simulink library "GTMLE_Library"  (R2014a)
settings: Solver=ode45  StartTime=0.0  StopTime=10.0  RelTol=1e-3
undefined symbols (not defined in the file or in its folder): CCP, DiscIntNeverNeededParam, DPos_test, sample_time, TData_test
undefined symbols (not defined in the file): MCP, steadydata
libraries: simulink x10, GTMLE_Library x2, discretizing x1
(part 1 of 2)
settings Model: CovSFcnEnable=on  Creator=Esrod  LastModifiedBy=Shubo

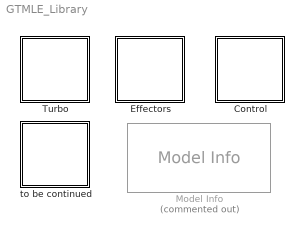
== system GTMLE_Library ==
  Control : Subsystem
  Effectors : Subsystem
  Model Info : simulink/Model-Wide Utilities/Model Info  Commented=on  InitialBlockCM=无  BlockCM=none  Frame=on  DisplayStringWithTags=|  HorizontalTextAlignment=Center  LeftAlignmentValue=0.5  SourceBlockDiagram=GTMLE_Library  TagMaxNumber=20
      | Model Info
      | %<ModifiedBy>
      | %<ModifiedDate>
      | %<ModifiedComment>
      | %<ModelVersion>
  Turbo : Subsystem
  to be continued : Subsystem

== system GTMLE_Library/Control ==
  ABControl : Subsystem  mask{CNST=CCP.CNST, PLA_TO=CCP.PLA_TO, PLA_MAX=CCP.PLA_MAX}
  Acc N1dot : Subsystem
  Acc Plan : Subsystem
  Static Control : Subsystem  mask{PLA_idle=CCP.PLA_idle, PLA_TO=CCP.PLA_TO, N1cor_TO=CCP.N1cor_TO*0.98, N1cor_idle=CCP.N1cor_idle}
  anti_windup : Subsystem

== system GTMLE_Library/Effectors ==
  DesignTools : Subsystem  InitFcn=load( 'resource/SS_Tool_result' );  mask{T4res=1700, SMres=20, n2_tab=steadydata(:,9), n2_Wfmin=steadydata(:,10)*0.7, kci=1e-4, accordec=2, statedata=[steadydata(:,10) steadydata(:,8) steadydata(:,9)]}
      mask prompts: T4res "T4resForAcc (K)"; SMres "SMresForAcc (%)"; n2_tab "n2_tab (rpm)"; n2_Wfmin "WfminForDec (kg/s)"; kci "kci (-)"; accordec "(1)ForAccPlan(2)ForDecPlan"
  Display_out : Subsystem
  Iterative NR Solver w JacobianCalc : Subsystem  mask(T-MATS: Iterative NR Solver w Jacobian Calc Library Block){SJac_Per_M=MCP.Solve.NR_Per_M(1:6,1), SNR_IC_M=MCP.Solve.NR_IC(1:6,1), SNR_DX_M=0.1, SJacobianAttempts_M=20, Cond_Limits_M=MCP.Solve.Cond_Limits_M}
      mask prompts: SJac_Per_M "SJac_Per_M - Jacobian Perturbation size (frac) (nx1)"; SNR_IC_M "SNR_IC_M - Newton Raphson Initial Conditions (nx1)"; SNR_DX_M "SNR_DX_M - Newton Raphson delta x limiter (%) (1x1)"; SJacobianAttempts_M "SJacobianAttempts_M - Newton Raphson attempts before the Jacobian recalculation (1x1)"; Cond_Limits_M "Cond_Limits_M - Iteration Conditions Limits (nx1 or 1x1)"
      mask help:
      | The Iterative Newton Raphson Solver with Jacobian Calculator block will
      | supply the inputs to iteratively drive the outputs of a system to zero.
      |
      | This will be performed in three steps.
      | 1) Jabobian calculator sends Perturbations to the plant then calculates the plant
      | Jacboian based on the system response
      | 2) The Newton Raphson will use the inverse of the Jacobian to iteratively step the
      | system toward solution.
      | 3) Once the solution has satisfied the conditions the Newton Raphson is shut off.
      |
      | This module is designed for dynamic systems and should be paired with
      | a "do... while" block in Simulink. The "do...while" block and this module
      | should both be located in the same subsystem as the plant that is to be solved for.
      mask Help: web(which('Solver_TMATS_INRSwJC.html'),'-helpbrowser')
  LoadTestData : Subsystem  mask{TData_test=TData_test, DPos_test=DPos_test}
  Mixer_Ades_calc : Subsystem  mask{Mades1=0.4, Mades2=0.451238}
      mask prompts: Mades1 "Core entry Mach in design condition"; Mades2 "Duct entry Mach in design condition"
  Performance : Subsystem
  SStool : Subsystem  StopFcn=|  mask{Wf_init=1.279, Wf_plan=[1 0.9 0.8 0.6 0.5 0.15], Cond_Limits_M=0.00001}
      | steadydata = importdata( 'resource/SS_Tool_Result.txt' );
      | save resource/SS_Tool_Result steadydata;                 
      | clearvars steadydata;                                    
      | delete( 'resource/SS_Tool_Result.txt' );

== system GTMLE_Library/Turbo ==
  Ambient : Subsystem
  Burner : Subsystem  mask(GTML_E: Burner Library Block){Eff_des=MCP.Buner.Eff_des, dpbur=MCP.Buner.dpbur, PtIn_des=MCP.Buner.PtIn_des, WIn_des=MCP.Buner.WIn_des, TtIn_des=MCP.Buner.TtIn_des, Volume=0.03, FuelType=Kerosene, TtIn_fuel=MCP.Buner.TtIn_fuel, LHV=MCP.Buner.LHV, FixEff=Constant Efficiency, CNST=MCP.Buner.CNST, Load_tab=MCP.Buner.Load_tab, Eff_tab=MCP.Buner.Eff_tab}
      mask prompts: Eff_des "Eff - Burner Efficiency"; dpbur "dpbur - Normalized Burner deltaP"; PtIn_des "<PtIn_des:kPa> - PtIn in design condition"; WIn_des "<WIn_des:kg/s> - WtIn in design condition"; TtIn_des "<TtIn_des:K> - TtIn in design condition"; Volume "Volume: m^3"; FuelType "Fuel type"; TtIn_fuel "<TtIn_fuel:K>"; LHV "<LHV:J/kg> - Fuel Lower Heating Value"; FixEff "Constant combustion efficiency"; Load_tab "Table of combustion load"; Eff_tab "Table of combustion efficiency"
      mask help: This block simulates the performance of a burner using basic thermodynamic equations and properties.
      mask TypeOptions FuelType: Kerosene | Nature Gas
      mask TypeOptions FixEff: Constant Efficiency | Using Characteristic Map
  Compressor : Subsystem  mask{CNST=MCP.Comp.CNST, N_tab=MCP.Comp.N_tab, Beta_tab=MCP.Comp.Beta_tab, Pi_tab=MCP.Comp.Pi_tab, Wcor_tab=MCP.Comp.Wcor_tab, Eta_tab=MCP.Comp.Eta_tab, CustBldsPlan=[0;0;0], FBldsPlan=[0;0;0], WcSurgeVec=MCP.Comp.WcSurgeVec, PRSurgeVec=MCP.Comp.PRSurgeVec}
  Duct : Subsystem  mask(Untitled: Duct Library Block){CNST=[101.325 288.15], sigma_des=0.8688, PtIn_des=292.164, WIn_des=35.22685, TtIn_des=430.59982}
      mask prompts: sigma_des "sigma_des - Rel. total pressure recovery coefficient"; PtIn_des "PtIn_des - PtIn in design condition"; WIn_des "WIn_des - WIn in design condition"; TtIn_des "TtIn_des - TtIn in design condition"
      mask help: This block simulates the performance of a duct using basic fluid dynamic equations and properties.
  Fan : Subsystem  mask{BPRdes=5.05, Cf=0}
  Heat Soakage : Subsystem  VariantControl=Variant1  mask(Heat Soakage){FCdes=MCP.Hpt.FC_des, Cpdes=MCP.Hpt.Cp_des, Wdes=MCP.Hpt.W_des, Aht=MCP.Hpt.Aht, Ck=MCP.Hpt.Ck, Mm=MCP.Hpt.Mm, Cm=MCP.Hpt.Cm, Ct=MCP.Hpt.Ct, x=MCP.Hpt.x}
      mask prompts: FCdes "FCdes[W/m^2 K]--Film coefficient"; Cpdes "Cpdes[J/kg K]--The gas specific heat in the design point"; Wdes "Wdes[kg/s]--Mass flow in the design point"; Aht "Aht[m^2]--Effective contact surface"; Ck "Ck[-] --A corrected factor for K"; Mm "Mm[kg]--Material effective mass"; Cm "Cm[J/kg K]--Material specific heat component material"; Ct "Ct[-]--A corrected factor for Tau"; x "x[-]--power,0~1"
      mask help:
      | K = Ck * FCdes * Aht * W^(x-1) / Cpdes / Wdes^x
      | Tau_inv = Ct * K * W * Cp / Cm / Mm
      | where Ct and Ck are corrected factors.
      | dTm/dt = Tau_inv * (Tg_ideal - Tm)
      | Tg_real = (1-K) * Tg_ideal + K * Tm
      mask Help:
      | Uht = 1/((1/FC)+(leff/km)) = FC when material thermal conductivity is not taken into account.
      | The material temperature dynamic response is a 1st order response following the equation:
      | 
      | Q =  Uht*Aht*(Tg_ideal-Tm)
      | 
      | FC is the film coefficient, calculated from
      | 
      | FC = FCdes*Cp/CPdes * (W/Wdes)^x
      | 
      | with FCdes as a user specified film coefficient in the design point. Cpdes and
      | Wdes are the gas specific heat and mass flow calculated for DP and Cp and
      | W the OD calculated values.
      | x = 0~1.
      | The average material temperature Tm is calculated by integrating:
      | 
      | dTm/dt = Q / (Cm*Mm)
      | 
      | Initial value for Tm is the steady state gas temperature. Since heat flow is
      | assumed to be proportional to the difference between gas and material temperature
      | the material temperature Tm follows the gas temperature Tg_ideal with a first
      | order lag.
      | The time constant is determined by:
      | 
      | Tau = Cm*Mm / (Uht*Aht)
      | 
      | The real gas temperature Tg_real is calculated by:
      | 
      | Tg_real = Tg_ideal - Q/W*Cp = (1-K) * Tg_ideal + K * Tm
      | 
      | with K = Ck * Uhtdes * Aht * W^(x-1) / Cpdes / Wdes^x
      | 
      | Symbols ---------- Description --------------------------------  Parameter name
      | Tm --------------- average material temperature
      | Tg_real --------------- average gas temperature
      | Aht -------------- effective contact surface -------------- Heat soak A
      | Cm --------------- specific heat component material ------- Heat soak Cp
      | Mm --------------- Effective mass ------------------------- Heat soak mass
      | Uht -------------- Heat transfer coefficient -------------- Uhsoak
      | Leff ------------- effective length heat flow transport --- Heat soak Leff
      | km --------------- material thermal conductivity ---------- Heat soak k
      | FC --------------- Film coefficient ----------------------- Heat soak film coefficient
      | W ---------------- Gas mass flow
      | Cp --------------- Gas specific heat
  Inlet : Subsystem  mask{sigma_inlet_des=MCP.Inlet.sigma}
  Mixer : Subsystem  mask(GTML_E: Mixer Library Block){Ades1=0.16, Ades2=0.18}
      mask prompts: Ades1 "<Acore_des:m^2> - Design core area"; Ades2 "<Aduct_des:m^2> - Design duct area"
      mask help: This block simulates the performance of a mixer.
  Nozzle : Subsystem  mask{CD=MCP.Ductnozzle.CD, CV=MCP.Ductnozzle.CV, CX=MCP.Ductnozzle.CX}
  Shaft : Subsystem  mask{J=MCP.Lowshaft.J, eta=MCP.Lowshaft.eta}
      mask prompts: J "<J:kg*m^2>"; eta "<ETAmech:->"
  Turbine : Subsystem  mask{CNST=MCP.Hpt.CNST, N_tab=MCP.Hpt.N_tab, Pi_tab=MCP.Hpt.Pi_tab, Wcor_tab=MCP.Hpt.Wcor_tab, Eta_tab=MCP.Hpt.Eta_tab, CoolingPlan=MCP.Hpt.CoolingPlan, FuelType=Kerosene}
      mask prompts: FuelType "Fuel type"
      mask TypeOptions FuelType: Kerosene | Nature Gas

== system GTMLE_Library/to be continued ==

== system GTMLE_Library/Control/ABControl ==
  PLA : Inport
  P2 : Inport  Port=2
  T2 : Inport  Port=3
  Divide : Product  Inputs=*/
  PLA_MAX : Constant  Value=PLA_MAX
  PLA_TO : Constant  Value=PLA_TO
  Product : Product
  Saturation : Saturate  UpperLimit=CCP.PLA_MAX  LowerLimit=CCP.PLA_TO
  Subsystem : Subsystem
  Sum : Sum  Inputs=|+-
  Sum1 : Sum  Inputs=|-+
  Wf_max : Constant  Value=CCP.AB.Wf_max
  Wf_ab : Outport
  wires:
  Saturation/1 -> Sum/1
  Wf_max/1 -> Subsystem/1(Wfmax)
  T2/1 -> Subsystem/3(T2)
  P2/1 -> Subsystem/2(P2)
  Subsystem/1(Wfmaxcor) -> Product/2
  Product/1 -> Wf_ab/1
  Divide/1 -> Product/1
  Sum1/1 -> Divide/2
  Sum/1 -> Divide/1
  PLA_MAX/1 -> Sum1/2
  PLA_TO/1 -> Sum/2, Sum1/1
  PLA/1 -> Saturation/1

== system GTMLE_Library/Control/Acc N1dot ==
  N1 : Inport
  Flag : Inport  Port=2
  Wf_initial : Inport  Port=3
  P2 : Inport  Port=4
  T2 : Inport  Port=5
  N2 : Inport  Port=6
  PI1 : Subsystem
  throttle plan : Subsystem
  WF_acc : Outport
  wires:
  N1/1 -> PI1/3(N1)
  T2/1 -> PI1/6(T2), throttle plan/3(T2)
  P2/1 -> PI1/5(P2), throttle plan/2(P2)
  Wf_initial/1 -> PI1/4(Wf_initial)
  N2/1 -> throttle plan/1(N2)
  Flag/1 -> PI1/2(Flag)
  throttle plan/1(" err_N2dot") -> PI1/1(y)
  PI1/1(Wf ndot) -> WF_acc/1

== system GTMLE_Library/Control/Acc Plan ==
  Ps3 : Inport
  N2 : Inport  Port=2
  T2 : Inport  Port=3
  1-D Lookup Table : Lookup_n-D  NumberOfTableDimensions=1  BreakpointsForDimension1=CCP.AccPlan.N2cor_Tab  Table=CCP.AccPlan.Wfcor_Tab  RndMeth=Simplest  InputSameDT=on
  Divide : Product  Inputs=*/
  Gain : Gain  Gain=1e-3
  Product : Product  RndMeth=Zero
  Product1 : Product  RndMeth=Zero
  a : Fcn  Expr=sqrt(288.15/u(1))
  Wfacc : Outport
  wires:
  1-D Lookup Table/1 -> Divide/1
  N2/1 -> Product/1
  Gain/1 -> Product1/2
  Product1/1 -> Wfacc/1
  Ps3/1 -> Gain/1  "kPa"
  Divide/1 -> Product1/1
  Product/1 -> 1-D Lookup Table/1
  a/1 -> Divide/2, Product/2
  T2/1 -> a/1

== system GTMLE_Library/Control/Static Control ==
  N1 : Inport
  PLA : Inport  Port=2
  T2 : Inport  Port=3
  P2 : Inport  Port=4
  Wf_initial : Inport  Port=5
  Flag : Inport  Port=6
  " " : Subsystem
  Display : Display
  Display1 : Display
  N1_cor : Subsystem
  Subsystem : Subsystem
  Sum : Sum  Inputs=|+-  SaturateOnIntegerOverflow=on
  Wfs : Outport
  wires:
  Flag/1 -> " "/6(Flag)
  Wf_initial/1 -> " "/5(Wf_initial)
  P2/1 -> " "/4(P2)
  T2/1 -> N1_cor/2(T2), " "/3(T2)
  PLA/1 -> Subsystem/1(PLA)
  Sum/1 -> " "/1(N1_eer)
  N1_cor/1(N1) -> Display/1, Sum/1
  Subsystem/1(N1cor) -> N1_cor/1(N1cor)
  " "/1(Wf) -> Wfs/1
  N1/1 -> Display1/1, " "/2(N1), Sum/2

== system GTMLE_Library/Control/anti_windup ==
  note: This block is for anti_windup.
      | Flag is for set point control, and the value of 1 represents to freeze the integral term, 0 to unfreeze the integral term.
      |  Flag2 is for acc. of N2dot control, and the value of 0 represents to freeze the integral term, 1 to unfreeze the integral term
      | Flag3 is for dec. of N2dot control, and the value of 0 represents to freeze the integral term, 1 to unfreeze the integral term
  set_point_Wf : Inport
  acc : Inport  Port=2
  acc_N2dot : Inport  Port=3
  dec : Inport  Port=4
  dec_N2dot : Inport  Port=5
  MinFcn : MATLAB Function  TreatAsAtomicUnit=on
  flag : Outport
  flag2 : Outport  Port=2
  Wf_above_idle : Outport  Port=3
  flag3 : Outport  Port=4
  wires:
  MinFcn/4(flag3) -> flag3/1
  MinFcn/2(flag) -> flag/1
  dec_N2dot/1 -> MinFcn/5(dec_N2dot)
  dec/1 -> MinFcn/3(dec)
  MinFcn/1(choose) -> Wf_above_idle/1
  MinFcn/3(flag2) -> flag2/1
  acc/1 -> MinFcn/2(acc)
  acc_N2dot/1 -> MinFcn/4(acc_N2dot)
  set_point_Wf/1 -> MinFcn/1(steady)

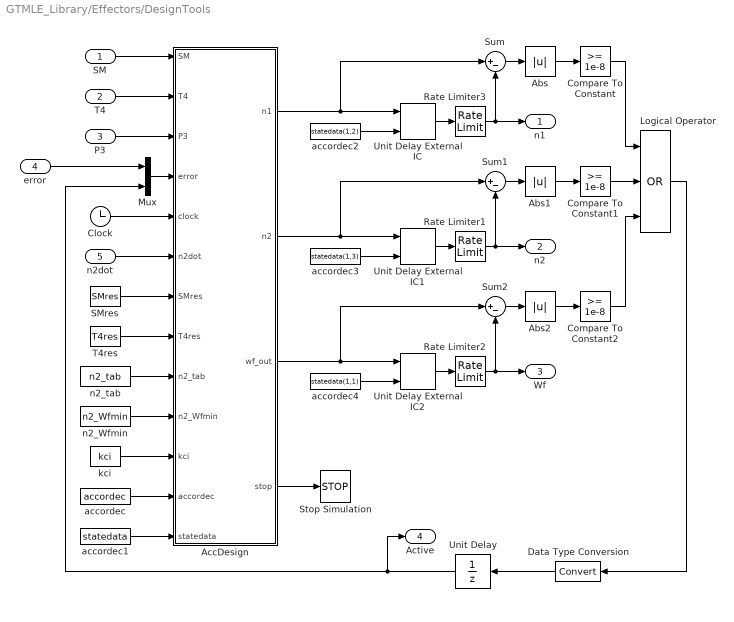
== system GTMLE_Library/Effectors/DesignTools ==
  SM : Inport
  T4 : Inport  Port=2
  P3 : Inport  Port=3
  error : Inport  Port=4
  n2dot : Inport  Port=5
  Abs : Abs
  Abs1 : Abs
  Abs2 : Abs
  AccDesign : MATLAB Function  TreatAsAtomicUnit=on
  Clock : Clock
  Compare To Constant : simulink/Logic and Bit Operations/Compare To Constant  relop=>=  const=1e-8  OutDataTypeStr=boolean
  Compare To Constant1 : simulink/Logic and Bit Operations/Compare To Constant  relop=>=  const=1e-8  OutDataTypeStr=boolean
  Compare To Constant2 : simulink/Logic and Bit Operations/Compare To Constant  relop=>=  const=1e-8  OutDataTypeStr=boolean
  Data Type Conversion : DataTypeConversion
  Logical Operator : Logic  Operator=OR  Inputs=3  AllPortsSameDT=off  OutDataTypeStr=boolean
  Mux : Mux  Inputs=2
  Rate Limiter1 : RateLimiter  RisingSlewLimit=10000  FallingSlewLimit=-10000  SampleTimeMode=inherited  InitialCondition=statedata(1,3)
  Rate Limiter2 : RateLimiter  RisingSlewLimit=2  FallingSlewLimit=-2  SampleTimeMode=inherited  InitialCondition=statedata(1,1)
  Rate Limiter3 : RateLimiter  RisingSlewLimit=10000  FallingSlewLimit=-10000  SampleTimeMode=inherited  InitialCondition=statedata(1,2)
  SMres : Constant  Value=SMres
  Stop Simulation : Stop
  Sum : Sum  Inputs=|+-
  Sum1 : Sum  Inputs=|+-
  Sum2 : Sum  Inputs=|+-
  T4res : Constant  Value=T4res
  Unit Delay : UnitDelay  InitialCondition=1  SampleTime=-1
  Unit Delay External IC : simulink/Additional Math & Discrete/Additional Discrete/Unit Delay External IC  tsamp=-1
  Unit Delay External IC1 : simulink/Additional Math & Discrete/Additional Discrete/Unit Delay External IC  tsamp=-1
  Unit Delay External IC2 : simulink/Additional Math & Discrete/Additional Discrete/Unit Delay External IC  tsamp=-1
  accordec : Constant  Value=accordec
  accordec1 : Constant  Value=statedata
  accordec2 : Constant  Value=statedata(1,2)
  accordec3 : Constant  Value=statedata(1,3)
  accordec4 : Constant  Value=statedata(1,1)
  kci : Constant  Value=kci
  n2_Wfmin : Constant  Value=n2_Wfmin
  n2_tab : Constant  Value=n2_tab
  n1 : Outport
  n2 : Outport  Port=2
  Wf : Outport  Port=3
  Active : Outport  Port=4
  wires:
  Data Type Conversion/1 -> Unit Delay/1
  Abs2/1 -> Compare To Constant2/1
  Abs1/1 -> Compare To Constant1/1
  Abs/1 -> Compare To Constant/1
  Unit Delay/1 -> Mux/2, Active/1
  Logical Operator/1 -> Data Type Conversion/1
  Mux/1 -> AccDesign/4(error)
  Compare To Constant2/1 -> Logical Operator/3
  Compare To Constant/1 -> Logical Operator/1
  Compare To Constant1/1 -> Logical Operator/2
  Sum2/1 -> Abs2/1
  AccDesign/3(wf_out) -> Unit Delay External IC2/1, Sum2/1
  Sum1/1 -> Abs1/1
  AccDesign/2(n2) -> Unit Delay External IC1/1, Sum1/1
  Sum/1 -> Abs/1
  Rate Limiter2/1 -> Wf/1, Sum2/2
  Rate Limiter1/1 -> n2/1, Sum1/2
  Rate Limiter3/1 -> n1/1, Sum/2
  accordec4/1 -> Unit Delay External IC2/2
  accordec3/1 -> Unit Delay External IC1/2
  accordec2/1 -> Unit Delay External IC/2
  Unit Delay External IC2/1 -> Rate Limiter2/1
  Unit Delay External IC1/1 -> Rate Limiter1/1
  Unit Delay External IC/1 -> Rate Limiter3/1
  accordec1/1 -> AccDesign/13(statedata)
  accordec/1 -> AccDesign/12(accordec)
  kci/1 -> AccDesign/11(kci)
  P3/1 -> AccDesign/3(P3)
  SM/1 -> AccDesign/1(SM)
  error/1 -> Mux/1
  T4/1 -> AccDesign/2(T4)
  Clock/1 -> AccDesign/5(clock)
  n2dot/1 -> AccDesign/6(n2dot)
  SMres/1 -> AccDesign/7(SMres)
  n2_tab/1 -> AccDesign/9(n2_tab)
  T4res/1 -> AccDesign/8(T4res)
  AccDesign/1(n1) -> Unit Delay External IC/1, Sum/1
  n2_Wfmin/1 -> AccDesign/10(n2_Wfmin)
  AccDesign/4(stop) -> Stop Simulation/1

== system GTMLE_Library/Effectors/Display_out ==
  input : Inport
  Abs : Abs
  Fcn : Fcn  Expr=(u(1)-u(2))/u(2)*100
  MinMax Running Resettable : simulink/Math Operations/MinMax Running Resettable  Function=max  vinit=0.0
  Scope1 : Outport
  Scope2 : Outport  Port=2
  Display : Outport  Port=3
  wires:
  input/1 -> Scope1/1, Fcn/1
  Abs/1 -> MinMax Running Resettable/1
  MinMax Running Resettable/1 -> Display/1
  Fcn/1 -> Abs/1, Scope2/1

== system GTMLE_Library/Effectors/Iterative NR Solver w JacobianCalc ==
  note: Note: During Building JC calc block will generally run before the plant, while the NR block will generally run after the plant
  Iterations : Inport
  Enable : Inport  Port=2
  f(x) : Inport  Port=3
  JC w Reset : Subsystem
  Logical Operator : Logic  AllPortsSameDT=off  OutDataTypeStr=boolean
  NRwCond : Subsystem
  do_while Condition : Outport
  X : Outport  Port=2
  S_Data : Outport  Port=3
  wires:
  f(x)/1 -> NRwCond/1(f(x)), JC w Reset/1(f(x))
  NRwCond/1(CCnd) -> Logical Operator/2
  Iterations/1 -> JC w Reset/2(Iter)
  NRwCond/2(y(n)) -> JC w Reset/3(y(n))
  JC w Reset/1(S_Data) -> S_Data/1
  JC w Reset/2(X_out) -> X/1
  JC w Reset/3(JC_Active) -> NRwCond/2(JC_Active)
  JC w Reset/4(inv(J)) -> NRwCond/3(inv(f'(x)))
  Enable/1 -> NRwCond/Enable, Logical Operator/1, JC w Reset/Enable
  Logical Operator/1 -> do_while Condition/1

== system GTMLE_Library/Effectors/LoadTestData ==
  clock : Inport
  Constant12 : Constant  Value=DPos_test
  Constant9 : Constant  Value=TData_test
  MATLAB Function4 : MATLAB Function  TreatAsAtomicUnit=on
  Data : Outport
  wires:
  MATLAB Function4/1(value) -> Data/1
  Constant12/1 -> MATLAB Function4/3(position_tab)
  Constant9/1 -> MATLAB Function4/2(value_tab)
  clock/1 -> MATLAB Function4/1(clock)

== system GTMLE_Library/Effectors/Mixer_Ades_calc ==
  GasPthCharIn_core : Inport
  GasPthCharIn_duct : Inport  Port=2
  Constant : Constant  Value=Mades1
  Constant1 : Constant  Value=Mades2
  MATLAB Function : MATLAB Function  TreatAsAtomicUnit=on
  <Ades1:m^2> : Outport
  <Ades2:m^2> : Outport  Port=2
  wires:
  MATLAB Function/2(Ades2) -> <Ades2:m^2>/1
  Constant1/1 -> MATLAB Function/4(Mades2)
  Constant/1 -> MATLAB Function/3(Mades1)
  GasPthCharIn_duct/1 -> MATLAB Function/2(GasPthCharIn2)
  MATLAB Function/1(Ades1) -> <Ades1:m^2>/1
  GasPthCharIn_core/1 -> MATLAB Function/1(GasPthCharIn1)

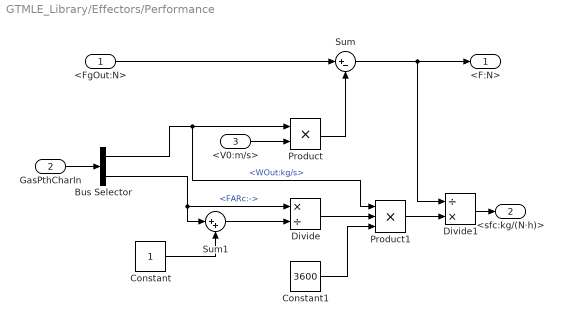
== system GTMLE_Library/Effectors/Performance ==
  <FgOut:N> : Inport
  GasPthCharIn : Inport  Port=2
  <V0:m/s> : Inport  Port=3
  Bus Selector : BusSelector  OutputSignals=WOut:kg/s,FARc:-
  Constant : Constant
  Constant1 : Constant  Value=3600
  Divide : Product  Inputs=*/
  Divide1 : Product  Inputs=/*
  Product : Product
  Product1 : Product  Inputs=3
  Sum : Sum  Inputs=|+-
  Sum1 : Sum  Inputs=|++
  <F:N> : Outport
  <sfc:kg/(N·h)> : Outport  Port=2
  wires:
  Divide1/1 -> <sfc:kg/(N·h)>/1
  Product1/1 -> Divide1/2
  Constant1/1 -> Product1/3
  Divide/1 -> Product1/2
  Constant/1 -> Sum1/2
  Sum1/1 -> Divide/2
  Bus Selector/2 -> Divide/1, Sum1/1  "<FARc:->"
  Bus Selector/1 -> Product/1, Product1/1  "<WOut:kg/s>"
  <V0:m/s>/1 -> Product/2
  Product/1 -> Sum/2
  GasPthCharIn/1 -> Bus Selector/1
  Sum/1 -> <F:N>/1, Divide1/1
  <FgOut:N>/1 -> Sum/1

== system GTMLE_Library/Effectors/SStool ==
  X : Inport
  Err : Inport  Port=2
  Active : UnitDelay  SampleTime=-1
  Compare To Zero : simulink/Logic and Bit Operations/Compare To Zero  relop===  OutDataTypeStr=boolean
  Constant1 : Constant  Value=Wf_init
  Constant5 : Constant  Value=Wf_plan
  Iteration Conditions : Subsystem
  Rate Limiter : RateLimiter  SampleTimeMode=inherited  InitialCondition=Wf_init
  Stop Simulation : Stop
  Sum : Sum  Inputs=|+-
  Wf_Schedule : MATLAB Function  TreatAsAtomicUnit=on
  cnt : UnitDelay  SampleTime=-1
  cnt1 : UnitDelay  InitialCondition=Wf_init  SampleTime=-1
  Wf : Outport
  wires:
  Iteration Conditions/1(Condition) -> Wf_Schedule/4(Err)
  Compare To Zero/1 -> Active/1
  Sum/1 -> Compare To Zero/1
  Wf_Schedule/3(Out_cnt) -> cnt/1
  Wf_Schedule/2(stop_flag) -> Stop Simulation/1
  X/1 -> Wf_Schedule/3(X)
  Err/1 -> Iteration Conditions/1(f(x))
  Rate Limiter/1 -> Wf/1, Sum/2
  cnt/1 -> Wf_Schedule/6(cnt)
  Active/1 -> Wf_Schedule/5(Active)
  cnt1/1 -> Rate Limiter/1
  Constant1/1 -> Wf_Schedule/1(Wf_init)
  Wf_Schedule/1(Out_Wf) -> Sum/1, cnt1/1
  Constant5/1 -> Wf_Schedule/2(Wf_plan)

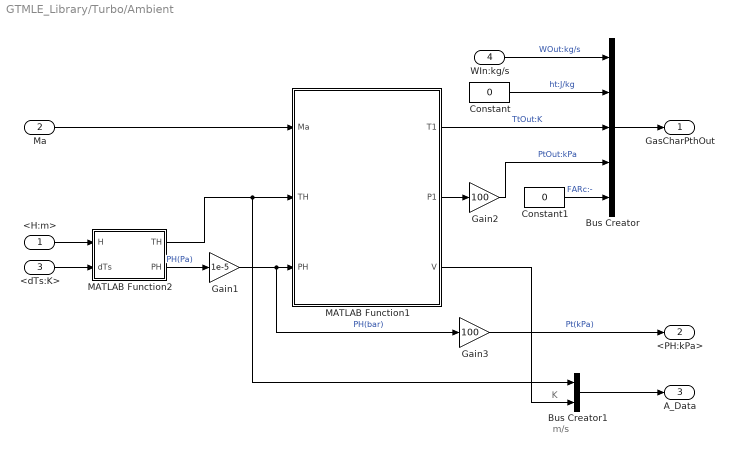
== system GTMLE_Library/Turbo/Ambient ==
  note: m/s
  note: K
  <H:m> : Inport
  Ma : Inport  Port=2
  <dTs:K> : Inport  Port=3
  WIn:kg/s : Inport  Port=4
  Bus Creator : BusCreator  Inputs=5
  Bus Creator1 : BusCreator  Inputs=2
  Constant : Constant  Value=0
  Constant1 : Constant  Value=0
  Gain1 : Gain  Gain=1e-5
  Gain2 : Gain  Gain=100
  Gain3 : Gain  Gain=100
  MATLAB Function1 : MATLAB Function  TreatAsAtomicUnit=on
  MATLAB Function2 : MATLAB Function  TreatAsAtomicUnit=on
  GasCharPthOut : Outport
  <PH:kPa> : Outport  Port=2
  A_Data : Outport  Port=3
  wires:
  WIn:kg/s/1 -> Bus Creator/1  "WOut:kg/s"
  Constant1/1 -> Bus Creator/5  "FARc:-"
  <dTs:K>/1 -> MATLAB Function2/2(dTs)
  MATLAB Function1/3(V) -> Bus Creator1/2
  Bus Creator1/1 -> A_Data/1
  Ma/1 -> MATLAB Function1/1(Ma)
  MATLAB Function1/2(P1) -> Gain2/1
  MATLAB Function1/1(T1) -> Bus Creator/3  "TtOut:K"
  <H:m>/1 -> MATLAB Function2/1(H)
  Gain1/1 -> Gain3/1, MATLAB Function1/3(PH)  "PH(bar)"
  Bus Creator/1 -> GasCharPthOut/1
  Constant/1 -> Bus Creator/2  "ht:J/kg"
  Gain2/1 -> Bus Creator/4  "PtOut:kPa"
  Gain3/1 -> <PH:kPa>/1  "Pt(kPa)"
  MATLAB Function2/1(TH) -> MATLAB Function1/2(TH), Bus Creator1/1
  MATLAB Function2/2(PH) -> Gain1/1  "PH(Pa)"

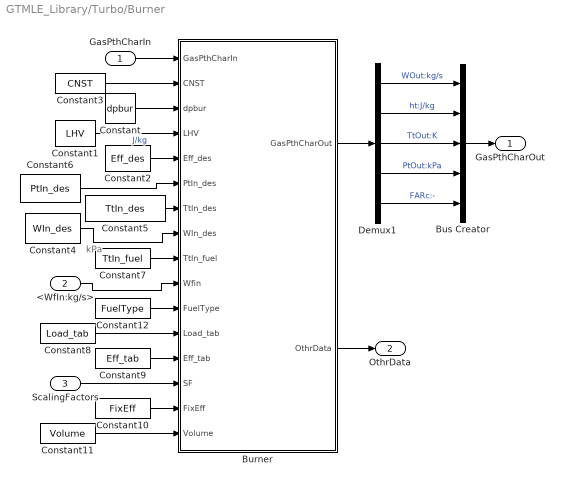
== system GTMLE_Library/Turbo/Burner ==
  note: kPa
  GasPthCharIn : Inport
  <WfIn:kg/s> : Inport  Port=2
  ScalingFactors : Inport  Port=3  PortDimensions=[2 1]
  Burner : MATLAB Function  TreatAsAtomicUnit=on
  Bus Creator : BusCreator  Inputs=5
  Constant : Constant  Value=dpbur
  Constant1 : Constant  Value=LHV
  Constant10 : Constant  Value=FixEff
  Constant11 : Constant  Value=Volume
  Constant12 : Constant  Value=FuelType
  Constant2 : Constant  Value=Eff_des
  Constant3 : Constant  Value=CNST
  Constant4 : Constant  Value=WIn_des
  Constant5 : Constant  Value=TtIn_des
  Constant6 : Constant  Value=PtIn_des
  Constant7 : Constant  Value=TtIn_fuel
  Constant8 : Constant  Value=Load_tab
  Constant9 : Constant  Value=Eff_tab
  Demux1 : Demux  Outputs=5
  GasPthCharOut : Outport
  OthrData : Outport  Port=2
  wires:
  Burner/2(OthrData) -> OthrData/1
  Constant11/1 -> Burner/16(Volume)
  Constant10/1 -> Burner/15(FixEff)
  Constant9/1 -> Burner/13(Eff_tab)
  Constant8/1 -> Burner/12(Load_tab)
  ScalingFactors/1 -> Burner/14(SF)
  Constant12/1 -> Burner/11(FuelType)
  Bus Creator/1 -> GasPthCharOut/1
  Burner/1(GasPthCharOut) -> Demux1/1
  Demux1/3 -> Bus Creator/3  "TtOut:K"
  Demux1/4 -> Bus Creator/4  "PtOut:kPa"
  Demux1/1 -> Bus Creator/1  "WOut:kg/s"
  Demux1/2 -> Bus Creator/2  "ht:J/kg"
  Demux1/5 -> Bus Creator/5  "FARc:-"
  <WfIn:kg/s>/1 -> Burner/10(Wfin)
  GasPthCharIn/1 -> Burner/1(GasPthCharIn)
  Constant3/1 -> Burner/2(CNST)
  Constant/1 -> Burner/3(dpbur)
  Constant1/1 -> Burner/4(LHV)  "J/kg"
  Constant2/1 -> Burner/5(Eff_des)
  Constant4/1 -> Burner/8(WIn_des)
  Constant6/1 -> Burner/6(PtIn_des)
  Constant5/1 -> Burner/7(TtIn_des)
  Constant7/1 -> Burner/9(TtIn_fuel)

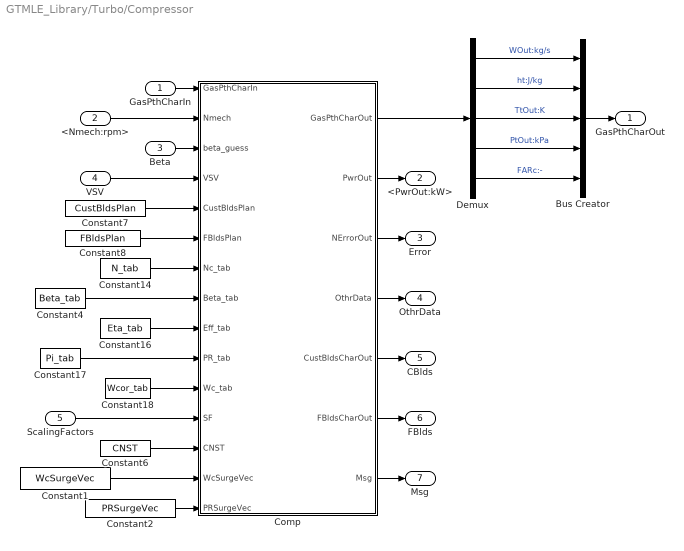
== system GTMLE_Library/Turbo/Compressor ==
  GasPthCharIn : Inport
  <Nmech:rpm> : Inport  Port=2
  Beta : Inport  Port=3
  VSV : Inport  Port=4
  ScalingFactors : Inport  Port=5  PortDimensions=[4 1]
  Bus Creator : BusCreator  Inputs=5
  Comp : MATLAB Function  TreatAsAtomicUnit=on
  Constant1 : Constant  Value=WcSurgeVec
  Constant14 : Constant  Value=N_tab
  Constant16 : Constant  Value=Eta_tab
  Constant17 : Constant  Value=Pi_tab
  Constant18 : Constant  Value=Wcor_tab
  Constant2 : Constant  Value=PRSurgeVec
  Constant4 : Constant  Value=Beta_tab  VectorParams1D=off
  Constant6 : Constant  Value=CNST
  Constant7 : Constant  Value=CustBldsPlan
  Constant8 : Constant  Value=FBldsPlan
  Demux : Demux  Outputs=5
  GasPthCharOut : Outport
  <PwrOut:kW> : Outport  Port=2
  Error : Outport  Port=3
  OthrData : Outport  Port=4
  CBlds : Outport  Port=5
  FBlds : Outport  Port=6
  Msg : Outport  Port=7
  wires:
  Comp/7(Msg) -> Msg/1
  Constant2/1 -> Comp/15(PRSurgeVec)
  Constant1/1 -> Comp/14(WcSurgeVec)
  Constant6/1 -> Comp/13(CNST)
  ScalingFactors/1 -> Comp/12(SF)
  Constant18/1 -> Comp/11(Wc_tab)
  Constant17/1 -> Comp/10(PR_tab)
  Constant16/1 -> Comp/9(Eff_tab)
  Constant4/1 -> Comp/8(Beta_tab)
  Constant14/1 -> Comp/7(Nc_tab)
  Constant8/1 -> Comp/6(FBldsPlan)
  Constant7/1 -> Comp/5(CustBldsPlan)
  VSV/1 -> Comp/4(VSV)
  Bus Creator/1 -> GasPthCharOut/1
  Comp/4(OthrData) -> OthrData/1
  Comp/6(FBldsCharOut) -> FBlds/1
  Comp/5(CustBldsCharOut) -> CBlds/1
  Comp/1(GasPthCharOut) -> Demux/1
  Demux/3 -> Bus Creator/3  "TtOut:K"
  Demux/4 -> Bus Creator/4  "PtOut:kPa"
  Comp/3(NErrorOut) -> Error/1
  Demux/1 -> Bus Creator/1  "WOut:kg/s"
  Demux/2 -> Bus Creator/2  "ht:J/kg"
  Demux/5 -> Bus Creator/5  "FARc:-"
  <Nmech:rpm>/1 -> Comp/2(Nmech)
  Beta/1 -> Comp/3(beta_guess)
  GasPthCharIn/1 -> Comp/1(GasPthCharIn)
  Comp/2(PwrOut) -> <PwrOut:kW>/1

== system GTMLE_Library/Turbo/Duct ==
  GasPthCharIn : Inport
  GasBlds : Inport  Port=2
  Bus Creator : BusCreator  Inputs=5
  Constant10 : Constant  Value=PtIn_des
  Constant12 : Constant  Value=sigma_des
  Constant3 : Constant  Value=CNST
  Constant8 : Constant  Value=WIn_des
  Constant9 : Constant  Value=TtIn_des
  Demux1 : Demux  Outputs=5
  Duct : MATLAB Function  TreatAsAtomicUnit=on
  GasPthCharOut : Outport
  OthrData : Outport  Port=2
  wires:
  Constant9/1 -> Duct/4(TtIn_des)
  Constant8/1 -> Duct/5(WIn_des)
  Constant10/1 -> Duct/3(PtIn_des)
  GasPthCharIn/1 -> Duct/1(GasPthCharIn)
  Bus Creator/1 -> GasPthCharOut/1
  Duct/1(GasPthCharOut) -> Demux1/1
  Demux1/3 -> Bus Creator/3
  Demux1/4 -> Bus Creator/4
  Demux1/1 -> Bus Creator/1  "WOut:kg/s"
  Demux1/2 -> Bus Creator/2  "ht:J/kg"
  Demux1/5 -> Bus Creator/5  "FARc:-"
  GasBlds/1 -> Duct/7(Blds)
  Constant3/1 -> Duct/2(CNST)
  Constant12/1 -> Duct/6(sigma_des)
  Duct/2(OthrData) -> OthrData/1

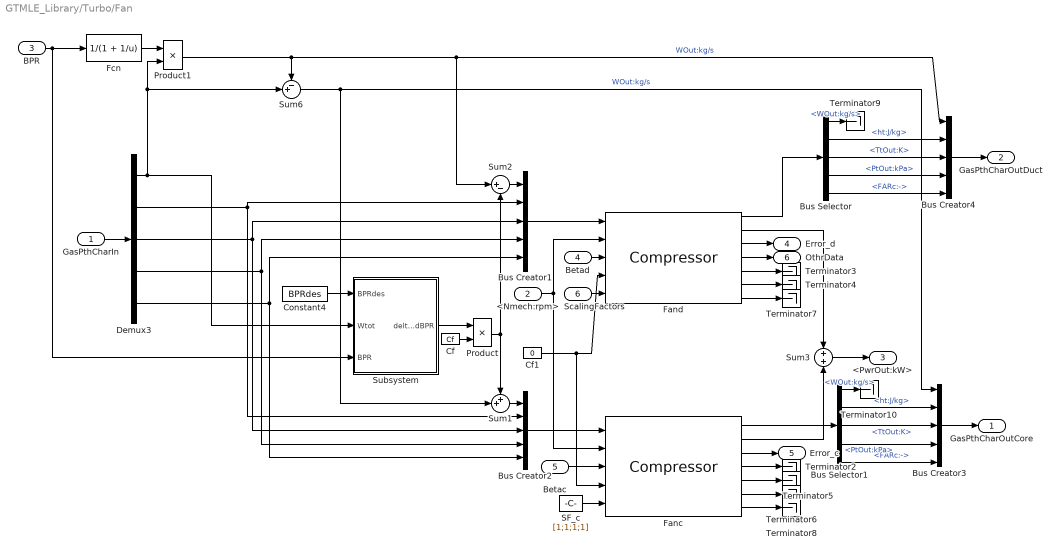
== system GTMLE_Library/Turbo/Fan ==
  GasPthCharIn : Inport
  <Nmech:rpm> : Inport  Port=2
  BPR : Inport  Port=3
  Betad : Inport  Port=4
  Betac : Inport  Port=5
  ScalingFactors : Inport  Port=6
  Bus Creator{1..4} (4 alike) : BusCreator  Inputs=5
  Bus Selector : BusSelector  OutputSignals=WOut:kg/s,ht:J/kg,TtOut:K,PtOut:kPa,FARc:-
  Bus Selector1 : BusSelector  OutputSignals=WOut:kg/s,ht:J/kg,TtOut:K,PtOut:kPa,FARc:-
  Cf : Constant  Value=Cf
  Cf1 : Constant  Value=0
  Constant4 : Constant  Value=BPRdes
  Demux3 : Demux  Outputs=5
  Fanc : GTMLE_Library/Turbo/Compressor  CNST=MCP.Fan.CNST  N_tab=MCP.Fan_core.N_tab  Beta_tab=MCP.Fan_core.Beta_tab  Pi_tab=MCP.Fan_core.Pi_tab  Wcor_tab=MCP.Fan_core.Wcor_tab  Eta_tab=MCP.Fan_core.Eta_tab  CustBldsPlan=[0;0;0]  FBldsPlan=[0;0;0]  WcSurgeVec=MCP.Fan_core.WcSurgeVec  PRSurgeVec=MCP.Fan_core.PRSurgeVec
  Fand : GTMLE_Library/Turbo/Compressor  CNST=MCP.Fan.CNST  N_tab=MCP.Fan_exduct.N_tab  Beta_tab=MCP.Fan_exduct.Beta_tab  Pi_tab=MCP.Fan_exduct.Pi_tab  Wcor_tab=MCP.Fan_exduct.Wcor_tab  Eta_tab=MCP.Fan_exduct.Eta_tab  CustBldsPlan=[0;0;0]  FBldsPlan=[0;0;0]  WcSurgeVec=MCP.Fan_exduct.WcSurgeVec  PRSurgeVec=MCP.Fan_exduct.PRSurgeVec
  Fcn : Fcn  Expr=1/(1 + 1/u)
  Product : Product
  Product1 : Product
  SF_c : Constant  Value=[1;1;1;1]
  Subsystem : Subsystem
  Sum1 : Sum  Inputs=++|
  Sum2 : Sum  Inputs=|+-
  Sum3 : Sum  Inputs=+|+
  Sum6 : Sum  Inputs=-+|
  Terminator{2..10} (9 alike) : Terminator
  GasPthCharOutCore : Outport
  GasPthCharOutDuct : Outport  Port=2
  <PwrOut:kW> : Outport  Port=3
  Error_d : Outport  Port=4
  Error_c : Outport  Port=5
  OthrData : Outport  Port=6
  wires:
  SF_c/1 -> Fanc/5
  ScalingFactors/1 -> Fand/5
  Fanc/4 -> Terminator2/1
  Fand/4 -> OthrData/1
  Demux3/1 -> Subsystem/2(Wtot), Product1/2, Sum6/2
  Bus Selector1/1 -> Terminator10/1  "<WOut:kg/s>"
  Bus Selector/1 -> Terminator9/1  "<WOut:kg/s>"
  Sum6/1 -> Sum1/2, Bus Creator3/1  "WOut:kg/s"
  Cf1/1 -> Fand/4, Fanc/4
  Fanc/7 -> Terminator8/1
  Fand/7 -> Terminator7/1
  Fand/3 -> Error_d/1
  Fanc/3 -> Error_c/1
  Fanc/6 -> Terminator6/1
  Betac/1 -> Fanc/3
  Betad/1 -> Fand/3
  Fanc/5 -> Terminator5/1
  Fand/6 -> Terminator4/1
  Fand/5 -> Terminator3/1
  Fcn/1 -> Product1/1
  BPR/1 -> Subsystem/3(BPR), Fcn/1
  Fand/1 -> Bus Selector/1
  Constant4/1 -> Subsystem/1(BPRdes)
  <Nmech:rpm>/1 -> Fand/2, Fanc/2
  Fanc/2 -> Sum3/2
  Demux3/3 -> Bus Creator1/3, Bus Creator2/3
  Demux3/4 -> Bus Creator1/4, Bus Creator2/4
  Product1/1 -> Sum2/1, Bus Creator4/1, Sum6/1  "WOut:kg/s"
  Fand/2 -> Sum3/1
  Bus Creator1/1 -> Fand/1
  Sum1/1 -> Bus Creator2/1
  Demux3/5 -> Bus Creator1/5, Bus Creator2/5
  Product/1 -> Sum1/1, Sum2/2
  Bus Creator2/1 -> Fanc/1
  Fanc/1 -> Bus Selector1/1
  Sum3/1 -> <PwrOut:kW>/1
  Demux3/2 -> Bus Creator1/2, Bus Creator2/2
  GasPthCharIn/1 -> Demux3/1
  Cf/1 -> Product/2
  Bus Selector1/5 -> Bus Creator3/5  "<FARc:->"
  Bus Selector/2 -> Bus Creator4/2  "<ht:J/kg>"
  Bus Selector1/3 -> Bus Creator3/3  "<TtOut:K>"
  Bus Selector/3 -> Bus Creator4/3  "<TtOut:K>"
  Bus Creator3/1 -> GasPthCharOutCore/1
  Subsystem/1(delta_mdBPR) -> Product/1
  Bus Selector1/4 -> Bus Creator3/4  "<PtOut:kPa>"
  Bus Selector/4 -> Bus Creator4/4  "<PtOut:kPa>"
  Bus Selector/5 -> Bus Creator4/5  "<FARc:->"
  Bus Selector1/2 -> Bus Creator3/2  "<ht:J/kg>"
  Bus Creator4/1 -> GasPthCharOutDuct/1
  Sum2/1 -> Bus Creator1/1

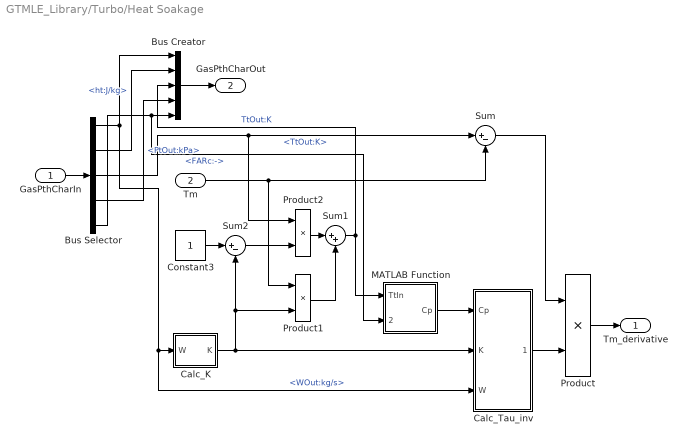
== system GTMLE_Library/Turbo/Heat Soakage ==
  GasPthCharIn : Inport
  Tm : Inport  Port=2
  Bus Creator : BusCreator  Inputs=5
  Bus Selector : BusSelector  OutputSignals=WOut:kg/s,ht:J/kg,TtOut:K,PtOut:kPa,FARc:-
  Calc_K : Subsystem
  Calc_Tau_inv : Subsystem
  Constant3 : Constant
  MATLAB Function : MATLAB Function  TreatAsAtomicUnit=on
  Product : Product
  Product1 : Product
  Product2 : Product
  Sum : Sum  Inputs=|+-
  Sum1 : Sum  Inputs=|++
  Sum2 : Sum  Inputs=|+-
  Tm_derivative : Outport
  GasPthCharOut : Outport  Port=2
  wires:
  Sum1/1 -> Bus Creator/3, MATLAB Function/1(TtIn)  "TtOut:K"
  Product/1 -> Tm_derivative/1
  Constant3/1 -> Sum2/1
  Sum2/1 -> Product2/2
  Calc_K/1(K) -> Product1/2, Sum2/2, Calc_Tau_inv/2(K)
  Calc_Tau_inv/1(Tau_inv) -> Product/2
  Sum/1 -> Product/1
  Bus Selector/3 -> Product2/1, Sum/1  "<TtOut:K>"
  Tm/1 -> Product1/1, Sum/2
  Product1/1 -> Sum1/2
  Product2/1 -> Sum1/1
  Bus Selector/1 -> Calc_Tau_inv/3(W), Calc_K/1(W), Bus Creator/1  "<WOut:kg/s>"
  Bus Selector/4 -> Bus Creator/4  "<PtOut:kPa>"
  Bus Selector/5 -> MATLAB Function/2(FARcIn), Bus Creator/5  "<FARc:->"
  Bus Creator/1 -> GasPthCharOut/1
  MATLAB Function/1(Cp) -> Calc_Tau_inv/1(Cp)
  Bus Selector/2 -> Bus Creator/2  "<ht:J/kg>"
  GasPthCharIn/1 -> Bus Selector/1

== system GTMLE_Library/Turbo/Inlet ==
  GasPthCharIn : Inport
  Bus Creator : BusCreator  Inputs=5
  Demux : Demux  Outputs=5
  Gain : Gain  Gain=sigma_inlet_des
  GasPthCharOut : Outport
  wires:
  Gain/1 -> Bus Creator/4  "PtOut:kPa"
  Demux/4 -> Gain/1
  GasPthCharIn/1 -> Demux/1
  Bus Creator/1 -> GasPthCharOut/1
  Demux/5 -> Bus Creator/5  "FARc:-"
  Demux/3 -> Bus Creator/3  "TtOut:K"
  Demux/2 -> Bus Creator/2  "ht:J/kg"
  Demux/1 -> Bus Creator/1  "WOut:kg/s"

== system GTMLE_Library/Turbo/Mixer ==
  GasPthCharCore : Inport
  GasPthCharDuct : Inport  Port=2
  Constant : Constant  Value=Ades1
  Constant1 : Constant  Value=Ades2
  Mixer : MATLAB Function  TreatAsAtomicUnit=on
  GasPthCharOut : Outport
  Error : Outport  Port=2
  <W2Calc:kg/s> : Outport  Port=3
  Msg : Outport  Port=4
  wires:
  Constant/1 -> Mixer/3(Adesign1)
  Constant1/1 -> Mixer/4(Adesign2)
  Mixer/1(GasPthCharOut) -> GasPthCharOut/1
  GasPthCharDuct/1 -> Mixer/2(GasPthCharIns)
  GasPthCharCore/1 -> Mixer/1(GasPthCharInp)
  Mixer/3(OthrData) -> <W2Calc:kg/s>/1
  Mixer/4(Msg) -> Msg/1
  Mixer/2(Error) -> Error/1

== system GTMLE_Library/Turbo/Nozzle ==
  GasPthCharIn : Inport
  <PambIn:kPa> : Inport  Port=2
  <AIn:m^2> : Inport  Port=3
  Constant1 : Constant  Value=CD
  Constant3 : Constant  Value=CX
  Constant5 : Constant  Value=CV
  Nozzle : MATLAB Function  TreatAsAtomicUnit=on
  <WOut:kg/s> : Outport
  <FgOut:N> : Outport  Port=2
  Error : Outport  Port=3
  OthrData : Outport  Port=4
  Msg : Outport  Port=5
  wires:
  Nozzle/4(OthrData) -> OthrData/1
  Nozzle/3(NErrorOut) -> Error/1
  Nozzle/2(FgOut) -> <FgOut:N>/1
  Nozzle/1(WOut) -> <WOut:kg/s>/1
  GasPthCharIn/1 -> Nozzle/1(GasPthCharIn)
  <PambIn:kPa>/1 -> Nozzle/2(PambIn)
  Constant3/1 -> Nozzle/6(CX)
  Constant5/1 -> Nozzle/5(CV)
  Constant1/1 -> Nozzle/4(Cdth)
  <AIn:m^2>/1 -> Nozzle/3(AthroatIn)
  Nozzle/5(Msg) -> Msg/1

== system GTMLE_Library/Turbo/Shaft ==
  <PowerC:kW> : Inport
  <PowerT:kW> : Inport  Port=2
  <Nmech:rpm> : Inport  Port=3
  Divide1 : Product  Inputs=*/
  Gain1 : Gain  Gain=1/eta
  Gain3 : Gain  Gain=1000
  Gain4 : Gain  Gain=(pi/30)^2
  J : Constant  Value=J
  Mux : Mux  Inputs=2
  Product1 : Product
  Sum of Elements : Sum  Inputs=+
  N_dot : Outport
  wires:
  Gain1/1 -> Mux/2
  <PowerT:kW>/1 -> Mux/1
  Mux/1 -> Sum of Elements/1
  <PowerC:kW>/1 -> Gain1/1
  Product1/1 -> Gain4/1
  Sum of Elements/1 -> Gain3/1
  Gain3/1 -> Divide1/1
  Gain4/1 -> Divide1/2
  J/1 -> Product1/2
  Divide1/1 -> N_dot/1
  <Nmech:rpm>/1 -> Product1/1

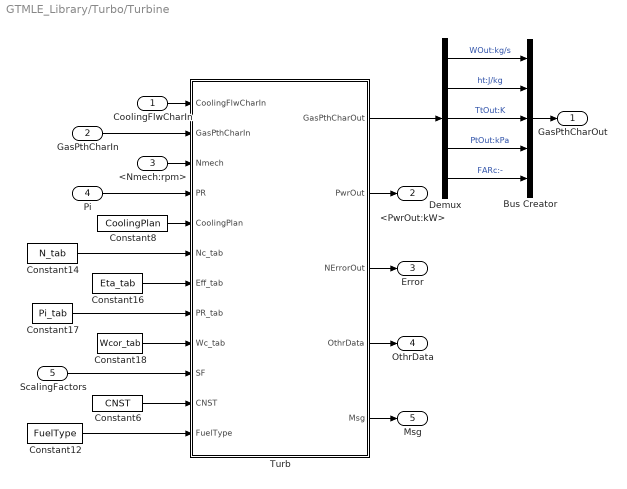
== system GTMLE_Library/Turbo/Turbine ==
  CoolingFlwCharIn : Inport
  GasPthCharIn : Inport  Port=2
  <Nmech:rpm> : Inport  Port=3
  Pi : Inport  Port=4
  ScalingFactors : Inport  Port=5  PortDimensions=[4 1]
  Bus Creator : BusCreator  Inputs=5
  Constant12 : Constant  Value=FuelType
  Constant14 : Constant  Value=N_tab
  Constant16 : Constant  Value=Eta_tab
  Constant17 : Constant  Value=Pi_tab
  Constant18 : Constant  Value=Wcor_tab
  Constant6 : Constant  Value=CNST
  Constant8 : Constant  Value=CoolingPlan
  Demux : Demux  Outputs=5
  Turb : MATLAB Function  TreatAsAtomicUnit=on
  GasPthCharOut : Outport
  <PwrOut:kW> : Outport  Port=2
  Error : Outport  Port=3
  OthrData : Outport  Port=4
  Msg : Outport  Port=5
  wires:
  Turb/5(Msg) -> Msg/1
  <Nmech:rpm>/1 -> Turb/3(Nmech)
  Turb/4(OthrData) -> OthrData/1
  Turb/3(NErrorOut) -> Error/1
  Constant14/1 -> Turb/6(Nc_tab)
  GasPthCharIn/1 -> Turb/2(GasPthCharIn)
  Constant8/1 -> Turb/5(CoolingPlan)
  ScalingFactors/1 -> Turb/10(SF)
  Constant18/1 -> Turb/9(Wc_tab)
  CoolingFlwCharIn/1 -> Turb/1(CoolingFlwCharIn)
  Pi/1 -> Turb/4(PR)
  Constant16/1 -> Turb/7(Eff_tab)
  Constant17/1 -> Turb/8(PR_tab)
  Constant6/1 -> Turb/11(CNST)
  Turb/2(PwrOut) -> <PwrOut:kW>/1
  Bus Creator/1 -> GasPthCharOut/1
  Turb/1(GasPthCharOut) -> Demux/1
  Demux/3 -> Bus Creator/3  "TtOut:K"
  Demux/4 -> Bus Creator/4  "PtOut:kPa"
  Demux/1 -> Bus Creator/1  "WOut:kg/s"
  Demux/2 -> Bus Creator/2  "ht:J/kg"
  Demux/5 -> Bus Creator/5  "FARc:-"
  Constant12/1 -> Turb/12(FuelType)

== system GTMLE_Library/Control/ABControl/Subsystem ==
  Wfmax : Inport
  P2 : Inport  Port=2
  T2 : Inport  Port=3
  Constant : Constant  Value=CNST
  Demux : Demux  Outputs=2
  Divide : Product  Inputs=*/
  Divide1 : Product  Inputs=/*
  Product : Product  Inputs=3
  Sqrt : Sqrt  SaturateOnIntegerOverflow=on
  Wfmaxcor : Outport
  wires:
  Product/1 -> Wfmaxcor/1
  Sqrt/1 -> Product/3
  Divide/1 -> Product/2
  Divide1/1 -> Sqrt/1
  Demux/2 -> Divide1/1
  T2/1 -> Divide1/2
  Demux/1 -> Divide/2
  P2/1 -> Divide/1
  Constant/1 -> Demux/1
  Wfmax/1 -> Product/1

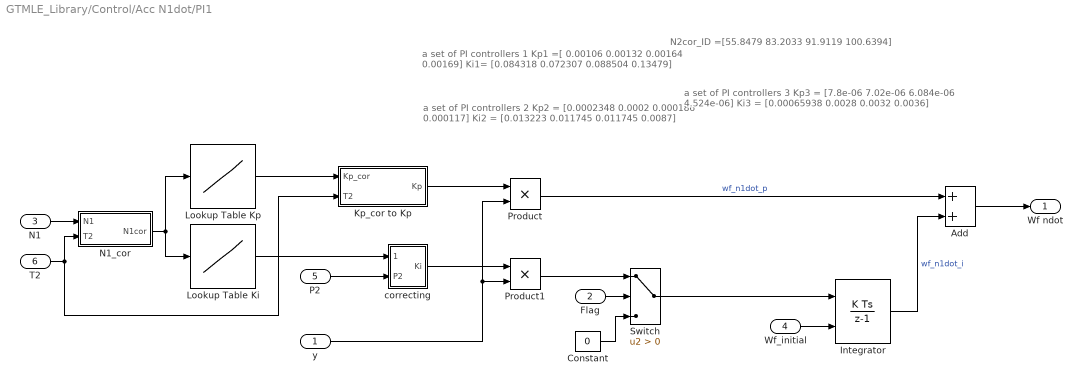
== system GTMLE_Library/Control/Acc N1dot/PI1 ==
  note: a set of PI controllers 1
      | Kp1 =[ 0.00106      0.00132      0.00164      0.00169]
      | Ki1= [0.084318     0.072307     0.088504      0.13479]
  note: N2cor_ID =[55.8479 83.2033 91.9119 100.6394]
  note: a set of PI controllers 2
      | Kp2 = [0.0002348       0.0002     0.000186     0.000117]
      | Ki2 = [0.013223     0.011745     0.011745       0.0087]
  note: a set of PI controllers 3
      | Kp3 = [7.8e-06     7.02e-06    6.084e-06    4.524e-06]
      | Ki3 = [0.00065938       0.0028       0.0032       0.0036]
  y : Inport
  Flag : Inport  Port=2
  N1 : Inport  Port=3
  Wf_initial : Inport  Port=4
  P2 : Inport  Port=5
  T2 : Inport  Port=6
  Add : Sum
  Constant : Constant  Value=0
  Integrator : DiscreteIntegrator  InitialConditionSource=external  SampleTime=sample_time  ICPrevOutput=DiscIntNeverNeededParam  ICPrevScaledInput=DiscIntNeverNeededParam  mask(DiscretizedDiscreteIntegrator){}
      mask init:
      | %tustin
  Kp_cor to Kp : Subsystem
  Lookup Table Ki : Lookup  InputValues=CCP.Ndot.N1cor_Tab  Table=CCP.Ndot.Ki_Tab
  Lookup Table Kp : Lookup  InputValues=CCP.Ndot.N1cor_Tab  Table=CCP.Ndot.Kp_Tab
  N1_cor : Subsystem
  Product : Product
  Product1 : Product
  Switch : Switch  Criteria=u2 > Threshold
  correcting : Subsystem
  Wf ndot : Outport
  wires:
  Kp_cor to Kp/1(Kp) -> Product/1
  Switch/1 -> Integrator/1
  T2/1 -> Kp_cor to Kp/2(T2), N1_cor/2(T2)
  P2/1 -> correcting/2(P2)
  correcting/1(Ki) -> Product1/1
  Lookup Table Ki/1 -> correcting/1(Kicor)
  Add/1 -> Wf ndot/1
  N1_cor/1(N1cor) -> Lookup Table Ki/1, Lookup Table Kp/1
  N1/1 -> N1_cor/1(N1)
  Product/1 -> Add/1  "wf_n1dot_p"
  Lookup Table Kp/1 -> Kp_cor to Kp/1(Kp_cor)
  Flag/1 -> Switch/2
  y/1 -> Product1/2, Product/2
  Integrator/1 -> Add/2  "wf_n1dot_i"
  Constant/1 -> Switch/3
  Product1/1 -> Switch/1
  Wf_initial/1 -> Integrator/2

== system GTMLE_Library/Control/Acc N1dot/throttle plan ==
  N2 : Inport
  P2 : Inport  Port=2
  T2 : Inport  Port=3
  Discrete Derivative : simulink/Discrete/Discrete Derivative  gainval=1.0  ICPrevScaledInput=0.0  InputProcessing=Inherited  OutMin=[]  OutMax=[]  OutDataType=fixdt(1, 16)  OutScaling=2^-10  DoSatur=off
  N2_cor : Subsystem
  N2dot_cor : Subsystem
  Ndot_acc : Lookup_n-D  NumberOfTableDimensions=1  BreakpointsForDimension1=CCP.AccPlan.N2cor_Tab  Table=CCP.AccPlan.N2dot_Tab  ExtrapMethod=Clip  RndMeth=Simplest  InputSameDT=on
  Saturation : Saturate  UpperLimit=1500  LowerLimit=-1500
  Scope : Scope
      settings: YMin=-10  YMax=10
  Sum : Sum  Inputs=|+-  SaturateOnIntegerOverflow=on
  Transfer Fcn : discretizing/Discretized Transfer Fcn  Numerator=[1]  Denominator=[0.01 1]  AbsTol=auto  SampleTime=sample_time  method=tustin  Wc=1
  " err_N2dot" : Outport
  wires:
  T2/1 -> N2dot_cor/2(P2)
  P2/1 -> N2_cor/2(T2)
  N2dot_cor/1(N2dot) -> Sum/1  "N2dot_cmd"
  Discrete Derivative/1 -> Saturation/1
  Transfer Fcn/1 -> Sum/2  "N2dot_sensor"
  N2/1 -> Discrete Derivative/1, N2_cor/1(N2)
  Ndot_acc/1 -> N2dot_cor/1(N2dotcor)
  Sum/1 -> " err_N2dot"/1, Scope/1  "N2dot_error"
  Saturation/1 -> Transfer Fcn/1
  N2_cor/1(N2cor) -> Ndot_acc/1

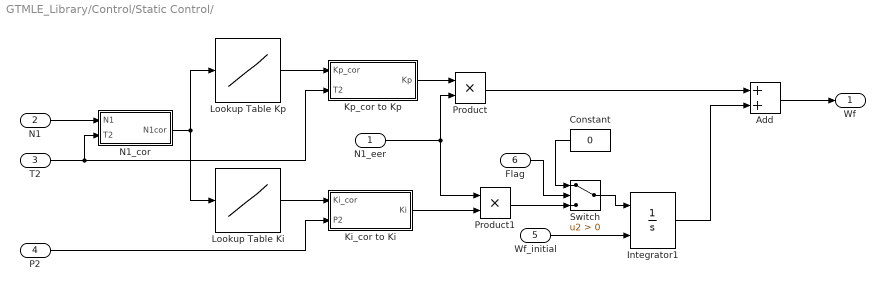
== system GTMLE_Library/Control/Static Control/  ==
  N1_eer : Inport
  N1 : Inport  Port=2
  T2 : Inport  Port=3
  P2 : Inport  Port=4
  Wf_initial : Inport  Port=5
  Flag : Inport  Port=6
  Add : Sum
  Constant : Constant  Value=0
  Integrator1 : Integrator  InitialConditionSource=external
  Ki_cor to Ki : Subsystem
  Kp_cor to Kp : Subsystem
  Lookup Table Ki : Lookup  InputValues=CCP.SC.N1cor_Tab  Table=CCP.SC.Ki_Tab
  Lookup Table Kp : Lookup  InputValues=CCP.SC.N1cor_Tab  Table=CCP.SC.Kp_Tab
  N1_cor : Subsystem
  Product : Product
  Product1 : Product
  Switch : Switch  Criteria=u2 > Threshold
  Wf : Outport
  wires:
  Flag/1 -> Switch/2
  Constant/1 -> Switch/1
  Switch/1 -> Integrator1/1
  P2/1 -> Ki_cor to Ki/2(P2)
  T2/1 -> N1_cor/2(T2), Kp_cor to Kp/2(T2)
  Product1/1 -> Switch/3
  Ki_cor to Ki/1(Ki) -> Product1/2
  Lookup Table Ki/1 -> Ki_cor to Ki/1(Ki_cor)
  Kp_cor to Kp/1(Kp) -> Product/1
  Lookup Table Kp/1 -> Kp_cor to Kp/1(Kp_cor)
  Wf_initial/1 -> Integrator1/2
  Add/1 -> Wf/1
  N1_cor/1(N1cor) -> Lookup Table Ki/1, Lookup Table Kp/1
  N1/1 -> N1_cor/1(N1)
  Product/1 -> Add/1
  N1_eer/1 -> Product1/1, Product/2
  Integrator1/1 -> Add/2

== system GTMLE_Library/Control/Static Control/N1_cor ==
  N1cor : Inport
  T2 : Inport  Port=2
  Mux4 : Mux  Inputs=2
  N1cor to N1 : Fcn  Expr=u(1)*sqrt(u(2)/288.15)
  N1 : Outport
  wires:
  Mux4/1 -> N1cor to N1/1
  T2/1 -> Mux4/2
  N1cor/1 -> Mux4/1
  N1cor to N1/1 -> N1/1

== system GTMLE_Library/Control/Static Control/Subsystem ==
  PLA : Inport
  Divide : Product  Inputs=*/
  N1cor_TO : Constant  Value=N1cor_TO
  N1cor_idle : Constant  Value=N1cor_idle
  PLA_TO : Constant  Value=PLA_TO
  PLA_idle : Constant  Value=PLA_idle
  Product : Product
  Saturation : Saturate  UpperLimit=CCP.PLA_TO  LowerLimit=CCP.PLA_idle
  Sum : Sum  Inputs=|+-
  Sum1 : Sum  Inputs=|-+
  Sum2 : Sum  Inputs=|+-
  Sum3 : Sum  Inputs=|++
  N1cor : Outport
  wires:
  Saturation/1 -> Sum/1
  Sum3/1 -> N1cor/1
  Product/1 -> Sum3/1
  Sum2/1 -> Product/2
  N1cor_idle/1 -> Sum3/2, Sum2/2
  N1cor_TO/1 -> Sum2/1
  Divide/1 -> Product/1
  Sum1/1 -> Divide/2
  Sum/1 -> Divide/1
  PLA_TO/1 -> Sum1/2
  PLA_idle/1 -> Sum/2, Sum1/1
  PLA/1 -> Saturation/1

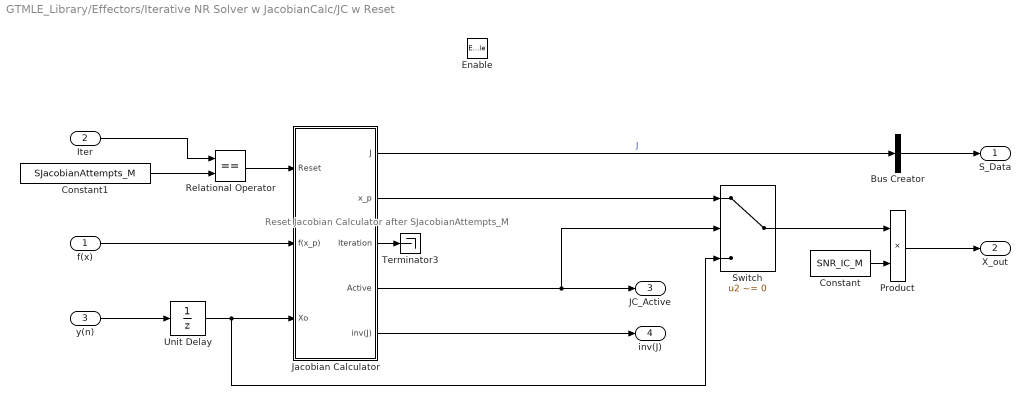
== system GTMLE_Library/Effectors/Iterative NR Solver w JacobianCalc/JC w Reset ==
  note: Reset Jacobian Calculator after SJacobianAttempts_M
  f(x) : Inport
  Iter : Inport  Port=2
  y(n) : Inport  Port=3
  Enable : EnablePort
  Bus Creator : BusCreator  Inputs=1
  Constant : Constant  Value=SNR_IC_M
  Constant1 : Constant  Value=SJacobianAttempts_M  OutDataTypeStr=uint32
  Jacobian Calculator : Subsystem  TreatAsAtomicUnit=on  mask(T-MATS: Jacobian Calculator Library Block){N_Per_M=SJac_Per_M}
      mask prompts: N_Per_M "N_Per_M - Perturbations (mx1)"
      mask help: The Jacobian Calculator block calculates the Jabobian of the system by perturbing the system around an initial point and calculating the gradient for each perturbation. This module will run once on start up and then again only if the reset is pressed and can operatewith m inputs, where m is the number of independents in the system.
      mask Help: web(which('NumMthd_TMATS_JC.html'),'-helpbrowser')
  Product : Product  RndMeth=Zero
  Relational Operator : RelationalOperator  Operator===  OutDataTypeStr=boolean
  Switch : Switch  Criteria=u2 ~= 0  Threshold=1
  Terminator3 : Terminator
  Unit Delay : UnitDelay  InitialCondition=ones(length(SNR_IC_M),1)  SampleTime=-1
  S_Data : Outport
  X_out : Outport  Port=2
  JC_Active : Outport  Port=3
  inv(J) : Outport  Port=4
  wires:
  f(x)/1 -> Jacobian Calculator/2(f(x_p))
  Jacobian Calculator/5(inv(J)) -> inv(J)/1
  Unit Delay/1 -> Switch/3, Jacobian Calculator/3(Xo)
  y(n)/1 -> Unit Delay/1
  Jacobian Calculator/1(J) -> Bus Creator/1  "J"
  Constant/1 -> Product/2
  Relational Operator/1 -> Jacobian Calculator/1(Reset)
  Product/1 -> X_out/1
  Jacobian Calculator/2(x_p) -> Switch/1
  Switch/1 -> Product/1
  Jacobian Calculator/4(Active) -> JC_Active/1, Switch/2
  Constant1/1 -> Relational Operator/2
  Iter/1 -> Relational Operator/1
  Bus Creator/1 -> S_Data/1
  Jacobian Calculator/3(Iteration) -> Terminator3/1

== system GTMLE_Library/Effectors/Iterative NR Solver w JacobianCalc/NRwCond ==
  note: Enable NR when conditions are not met
      | and Jacobian Calculator is not active
  f(x) : Inport
  JC_Active : Inport  Port=2
  inv(f'(x)) : Inport  Port=3
  Enable : EnablePort
  Iteration Conditions : Subsystem
  Logical Operator : Logic  Operator=NOT  AllPortsSameDT=off  OutDataTypeStr=boolean
  Logical Operator1 : Logic  AllPortsSameDT=off  OutDataTypeStr=boolean
  Newton Raphson Solver : Subsystem  TreatAsAtomicUnit=on  mask(T-MATS: Newton Raphson Solver Library Block){NR_IC_M=ones(length(SNR_IC_M),1), NR_dx_Lim_M=SNR_DX_M}
      mask prompts: NR_IC_M "NR_IC_M - Initial Conditions of Newton Raphson (mx1)"; NR_dx_Lim_M "NR_dx_Lim_M - Newton Raphson dx limit (%) (1x1)"
      mask help:
      | Newton Raphson Solver:
      |
      | x(n+1) = x(n) - inverse(f'(x(n)))*f(x(n))
      |
      | Note:
      | inverse(f'(x(n))) is an m x m matrix and f(x(n)) is an m x 1 matrix
      | where m is the length of the initial conditions matrix and number of system independents.
      mask Help: web(which('NumMthd_TMATS_NRS.html'),'-helpbrowser')
  Terminator : Terminator
  CCnd : Outport
  y(n) : Outport  Port=2
  wires:
  f(x)/1 -> Iteration Conditions/1(f(x)), Newton Raphson Solver/3(f(x(n)))
  JC_Active/1 -> Logical Operator/1
  Newton Raphson Solver/2(y(n)) -> y(n)/1
  Newton Raphson Solver/1(x(n+1)) -> Terminator/1
  inv(f'(x))/1 -> Newton Raphson Solver/2(inv(f'(x(n))))
  Logical Operator1/1 -> Newton Raphson Solver/1(Enable)
  Logical Operator/1 -> Logical Operator1/1
  Iteration Conditions/1(Condition) -> Logical Operator1/2, CCnd/1

== system GTMLE_Library/Effectors/SStool/Iteration Conditions ==
  f(x) : Inport
  Abs : Abs
  Constant1 : Constant  Value=Cond_Limits_M
  Constant2 : Constant  Value=0
  Relational Operator : RelationalOperator  Operator=>  OutDataTypeStr=boolean
  Relational Operator1 : RelationalOperator  Operator=>  OutDataTypeStr=boolean
  Sum of Elements : Sum  Inputs=+
  Condition : Outport
  wires:
  Abs/1 -> Relational Operator/1
  Constant1/1 -> Relational Operator/2
  f(x)/1 -> Abs/1
  Relational Operator/1 -> Sum of Elements/1
  Constant2/1 -> Relational Operator1/2
  Sum of Elements/1 -> Relational Operator1/1
  Relational Operator1/1 -> Condition/1

== system GTMLE_Library/Turbo/Fan/Subsystem ==
  BPRdes : Inport
  Wtot : Inport  Port=2
  BPR : Inport  Port=3
  Add1 : Sum
  Add2 : Sum
  Add3 : Sum  Inputs=-+
  Divide3 : Product  Inputs=*/
  Divide4 : Product  Inputs=*/
  Product : Product
  const : Constant
  const1 : Constant
  delta_mdBPR : Outport
  wires:
  BPR/1 -> Divide4/1, Add2/1
  Wtot/1 -> Product/2
  Product/1 -> delta_mdBPR/1
  Add3/1 -> Product/1
  Divide4/1 -> Add3/2
  Divide3/1 -> Add3/1
  Add2/1 -> Divide4/2
  const1/1 -> Add2/2
  Add1/1 -> Divide3/2
  const/1 -> Add1/2
  BPRdes/1 -> Divide3/1, Add1/1

== system GTMLE_Library/Turbo/Heat Soakage/Calc_K ==
  note: Station 4: 1220 16.247
  note: Station 3: 1087.2 19.960
  note: Station 31: 1087.2 15.844
  note: Station 41: 1208 19.333
  note: Station 45: 1156.1 20.671
  note: Station 5: 1078.8 21.238
  note: Cp_des-J/kg/K Wdes-kg/s
  note: K = Ck\timesFCdes\timesAht\timesW^{x-1} \div (Cp_{des}\timesWdes^{x})
  W : Inport
  Area : Constant  Value=Aht
  Cp_des : Constant  Value=Cpdes
  FCdes : Constant  Value=FCdes
  FCdes1 : Constant  Value=Ck
  FCdes2 : Constant  Value=x-1
  FCdes3 : Constant  Value=x
  Math Function : Math  Operator=pow  SaturateOnIntegerOverflow=on
  Math Function1 : Math  Operator=pow  SaturateOnIntegerOverflow=on
  Product : Product  Inputs=****//
  Wdes : Constant  Value=Wdes
  K : Outport
  wires:
  FCdes1/1 -> Product/1
  FCdes/1 -> Product/2  "FCdes"
  Area/1 -> Product/3  "A"
  W/1 -> Math Function/1
  FCdes2/1 -> Math Function/2
  Math Function/1 -> Product/4
  Cp_des/1 -> Product/5  "Cp_des"
  Product/1 -> K/1
  Wdes/1 -> Math Function1/1  "Wdes"
  FCdes3/1 -> Math Function1/2
  Math Function1/1 -> Product/6

== system GTMLE_Library/Turbo/Heat Soakage/Calc_Tau_inv ==
  note: Tau_{inv} = 1/\tau = Ct\timesCp\timesK\timesW \div (Mm\timesCm)
  Cp : Inport
  K : Inport  Port=2
  W : Inport  Port=3
  Cm : Constant  Value=Cm
  Ct : Constant  Value=Ct
  Product : Product  Inputs=****//
  m : Constant  Value=Mm
  Tau_inv : Outport
  wires:
  Product/1 -> Tau_inv/1
  Ct/1 -> Product/1
  Cp/1 -> Product/2
  K/1 -> Product/3
  W/1 -> Product/4
  Cm/1 -> Product/6
  m/1 -> Product/5

== system GTMLE_Library/Control/Acc N1dot/PI1/Kp_cor to Kp ==
  Kp_cor : Inport
  T2 : Inport  Port=2
  Fcn : Fcn  Expr=u(1)*sqrt(u(2)/288.15)
  Mux : Mux  Inputs=2
  Kp : Outport
  wires:
  Mux/1 -> Fcn/1
  T2/1 -> Mux/2
  Fcn/1 -> Kp/1
  Kp_cor/1 -> Mux/1

== system GTMLE_Library/Control/Acc N1dot/PI1/N1_cor ==
  N1 : Inport
  T2 : Inport  Port=2
  N1_cor : MATLAB Function  TreatAsAtomicUnit=on
  N1cor : Outport
  wires:
  T2/1 -> N1_cor/2(T2)
  N1_cor/1(N1cor) -> N1cor/1
  N1/1 -> N1_cor/1(N1)

== system GTMLE_Library/Control/Acc N1dot/PI1/correcting ==
  Kicor : Inport
  P2 : Inport  Port=2
  Fcn1 : Fcn  Expr=u(1)*(u(2)/101.325)
  Mux1 : Mux  Inputs=2
  Ki : Outport
  wires:
  P2/1 -> Mux1/2
  Fcn1/1 -> Ki/1
  Mux1/1 -> Fcn1/1
  Kicor/1 -> Mux1/1

== system GTMLE_Library/Control/Acc N1dot/throttle plan/N2_cor ==
  N2 : Inport
  T2 : Inport  Port=2
  Fcn : Fcn  Expr=(u(1)/sqrt(u(2)))*sqrt(288.15)
  Mux : Mux  Inputs=2
  N2cor : Outport
  wires:
  Mux/1 -> Fcn/1
  N2/1 -> Mux/1
  T2/1 -> Mux/2
  Fcn/1 -> N2cor/1

== system GTMLE_Library/Control/Acc N1dot/throttle plan/N2dot_cor ==
  N2dotcor : Inport
  P2 : Inport  Port=2
  Fcn1 : Fcn  Expr=u(1)*sqrt(u(2)/101.325)
  Mux : Mux  Inputs=2
  N2dot : Outport
  wires:
  Fcn1/1 -> N2dot/1
  Mux/1 -> Fcn1/1
  P2/1 -> Mux/2
  N2dotcor/1 -> Mux/1

== system GTMLE_Library/Control/Static Control/ /Ki_cor to Ki ==
  Ki_cor : Inport
  P2 : Inport  Port=2
  Fcn1 : Fcn  Expr=u(1)*u(2)/101.325
  Mux1 : Mux  Inputs=2
  Ki : Outport
  wires:
  Mux1/1 -> Fcn1/1
  P2/1 -> Mux1/2
  Fcn1/1 -> Ki/1
  Ki_cor/1 -> Mux1/1
